simulink model "P5_3_MatFunction"  (R2025b)
settings: Solver=VariableStepAuto  StartTime=0.0  StopTime=10.0  RelTol=1e-3
settings Model: Creator=tongx  LastModifiedBy=tongx

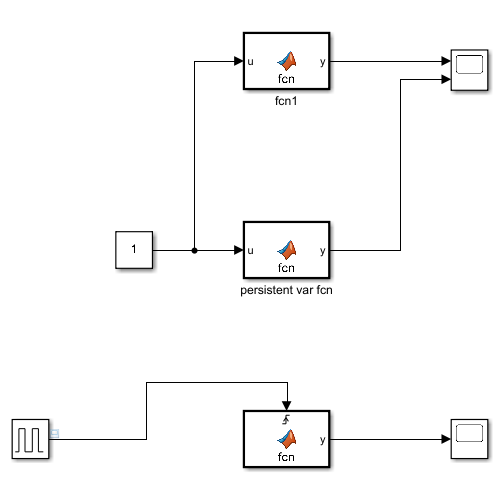
[thumbnail: Simulink's stored preview of the top-level diagram]
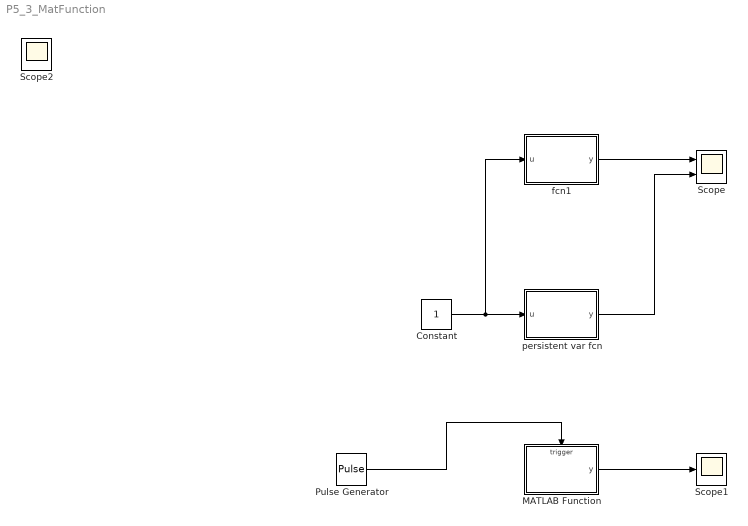
== system P5_3_MatFunction ==
  Constant : Constant
  MATLAB Function : MATLAB Function  TreatAsAtomicUnit=on
  Pulse Generator : DiscretePulseGenerator  PulseType=Time based  Period=1  PulseWidth=5
  Scope : Scope  NumInputPorts=2
      settings: ActiveDisplayYMinimum=-1  ActiveDisplayYMaximum=1
  Scope1 : Scope
      settings: ActiveDisplayYMinimum=-2.4999999999999996  ActiveDisplayYMaximum=22.5
  fcn1 : MATLAB Function  TreatAsAtomicUnit=on
  persistent var fcn : MATLAB Function  TreatAsAtomicUnit=on
  Scope2 : Scope
      settings: ActiveDisplayYMinimum=-0.12499999999999997  ActiveDisplayYMaximum=1.125  DataLoggingVariableName=ScopeData2
  wires:
  Constant/1 -> fcn1/1(u), persistent var fcn/1(u)
  persistent var fcn/1(y) -> Scope/2
  fcn1/1(y) -> Scope/1
  Pulse Generator/1 -> MATLAB Function/Trigger
  MATLAB Function/1(y) -> Scope1/1

== matlab function P5_3_MatFunction/persistent var fcn ==
  data: u input; y output
function y = fcn(u)

persistent x

if isempty(x)
    x = 0;
end

x = x + u;

y = x;

== matlab function P5_3_MatFunction/MATLAB Function ==
  data: y output
  events: trigger input RISING_EDGE_EVENT
function y = fcn()

persistent x

if isempty(x)
    x = 0;
end

x = x + 2;

y = x;

== matlab function P5_3_MatFunction/fcn1 ==
  data: u input; y output
function y = fcn(u)



y = u;
